simulink model "lane_dm6437_tcpip"  (Simulink 7.1)
settings: Solver=FixedStepDiscrete  SolverMode=SingleTasking  StartTime=0.0  StopTime=inf  RelTol=1e-3
PostLoadFcn:
  | NumRows=81
libraries: etargetslib x6, dspmtrx3 x2, viptransforms x2, dspindex x2, vipanalysis x1, vipobslib x1, dspstat3 x1, viptextngfix x1, vipstatistics x1, dspbioslib x1
CloseFcn:
  | clear vR3 vG3 vB3
settings Model: Creator=don  LastModifiedBy=Administrator
settings SolverCC: PositivePriorityOrder=on
settings DataIOCC: LimitDataPoints=off  SaveOutput=off  SaveTime=off  SignalLoggingName=sigsOut
settings OptimizationCC: EnforceIntegerDowncast=off  LocalBlockOutputs=off  OptimizeModelRefInitCode=on  BufferReusableBoundary=off
settings DebuggingCC: CheckExecutionContextPreStartOutputMsg=on  CheckExecutionContextRuntimeOutputMsg=on  SignalResolutionControl=TryResolveAllWithWarning  SolverPrmCheckMsg=none  MultiTaskDSMMsg=warning  MultiTaskCondExecSysMsg=none  SigSpecEnsureSampleTimeMsg=none
settings HardwareCC: ProdBitPerLong=40  ProdIntDivRoundTo=Zero  ProdEndianess=LittleEndian  ProdHWDeviceType=TI C6000  TargetHWDeviceType=32-bit Generic
settings ModelReferenceCC: UpdateModelReferenceTargets=IfOutOfDate
settings RTWCC: SystemTargetFile=ccslink_ert.tlc  GenerateMakefile=off  TemplateMakefile=ccslink_ert.tmf  Description=Embedded IDE Link CC (ERT) code generation for TMS320(TM) DSP platforms  ProcessScript=ccslink_ert_make_rtw_hook  IncludeERTFirstTime=on
settings CodeAppCC: IgnoreCustomStorageClasses=off
settings ERTTgtLinkCCS: TargetFcnLib=ansi_tfl_tmw_new.mat  TargetFunctionLibrary=ANSI_C  UtilityFuncGeneration=Auto  GenerateFullHeader=on  GenerateSampleERTMain=off  GenerateTestInterfaces=off  IsPILTarget=off  ModelReferenceCompliant=on  CompOptLevelCompliant=off  IncludeMdlTerminateFcn=on  CombineOutputUpdateFcns=on  SuppressErrorStatus=off  ERTFirstTimeCompliant=off  IncludeFileDelimiter=Auto  ERTCustomFileBanners=on  SupportAbsoluteTime=on  LogVarNameModifier=rt_  MatFileLogging=off  MultiInstanceERTCode=off  SupportNonFinite=on  SupportComplex=on  PurelyIntegerCode=off  SupportContinuousTime=off  SupportNonInlinedSFcns=off  EnableShiftOperators=on  ParenthesesLevel=Nominal  PortableWordSizes=off  ModelStepFunctionPrototypeControlCompliant=off  AutosarCompliant=off  GenerateErtSFunction=off  GenerateASAP2=off  ExtMode=off  ExtModeTransport=0  ExtModeStaticAlloc=on  ExtModeStaticAllocSize=1000000  ExtModeTesting=off  ExtModeMexFile=ext_comm  ExtModeIntrfLevel=Level1  InlinedParameterPlacement=NonHierarchical  TargetOS=BareBoardExample  MultiInstanceErrorCode=Error  RateGroupingCode=on  RootIOFormat=Individual arguments  RTWCAPISignals=off  RTWCAPIParams=off  RTWCAPIStates=off  ERTSrcFileBannerTemplate=ert_code_template.cgt  ERTHdrFileBannerTemplate=ert_code_template.cgt  ERTDataSrcFileTemplate=ert_code_template.cgt  ERTDataHdrFileTemplate=ert_code_template.cgt  ERTCustomFileTemplate=example_file_process.tlc  ModuleNamingRule=Unspecified  SignalDisplayLevel=10  ParamTuneLevel=10  GlobalDataDefinition=Auto  DataDefinitionFile=global.c  GlobalDataReference=Auto  DataReferenceFile=global.h  GRTInterface=off  PreserveExpressionOrder=off  PreserveIfCondition=off  EnableUserReplacementTypes=off  MemSecPackage=--- None ---  MemSecDataConstants=Default  MemSecDataIO=Default  MemSecDataInternal=Default  MemSecDataParameters=Default  MemSecFuncInitTerm=Default  MemSecFuncExecute=Default  exportIDEObj=on  ideObjName=CCS_Obj  oldideObjName=CCS_Obj  ideObjTimeout=10  oldideObjTimeout=10  ideObjBuildTimeout=1000  oldideObjBuildTimeout=1000  ProfileGenCode=off  ProfileNumSamples=100  InlineDSPBlks=on  projectOptions=Custom  debugCompilerOptions="-g -d\"_DEBUG\""  releaseCompilerOptions=-o2  customCompilerOptions=-o2 --mem_model:data=far  compilerOptionsStr=-o2 --mem_model:data=far  getCompilerOptions=off  getLinkerOptions=off  systemStackSize=8192  buildAction=Build  overrunNotificationMethod=None  overrunNotificationFcn=myfunction  oldoverrunNotificationFcn=myfunction  configurePIL=off  configPILBlockAction=None

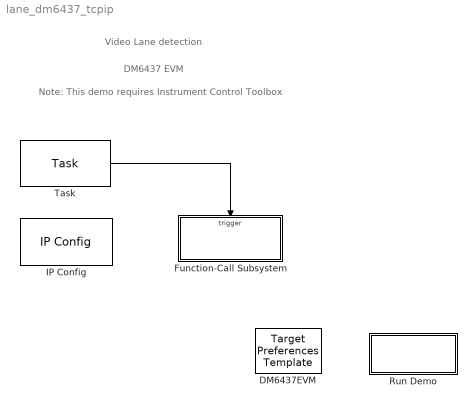
== system lane_dm6437_tcpip ==
  note: Video Lane detection
  note: DM6437 EVM
  note: Note: This demo requires Instrument Control Toolbox
  DM6437EVM : etargetslib/Target Preferences Template  Tag=ccslinktgtpref  SystemSampleTime=-1
  Function-Call Subsystem : Subsystem  TreatAsAtomicUnit=on
  IP Config : etargetslib/IP Config  boardType=DM6437EVM  daughterCard=Internal EMAC  tcpipStackDir=$(NDK_INSTALL_DIR)\packages\ti\ndk  enetIntNum=13  memSegment=DDR  enablePrintfs=on  dhcpEnabled=on  IPAddr=100.100.100.2  subnetMask=255.255.255.0  gatewayIP=100.100.100.1  dnsServerIP=0.0.0.0  domainName=mathworks.net  hostName=dm6437evm
  Run Demo : Subsystem  Description=Controls host-side RTDX processing.  AncestorBlock=demo_controls/Run Demo
      settings: OpenFcn=lane_tcpip_script('lane_pcl_tcpip');
      mask Display: disp(sprintf('Build / Reload\n& Run'))
  Task : dspbioslib/Task  SystemSampleTime=-1  taskName=Task0  taskPriority=1  taskExecutionOrder=1  taskStackSize=8192  stackMemSegment=IRAM  monitorStackUse=off  taskYield=off  parentmanaget=on  tickres=1/1000  ticklen=32bits  taskTrigger=off
  wires:
  Task/1 -> Function-Call Subsystem/Trigger

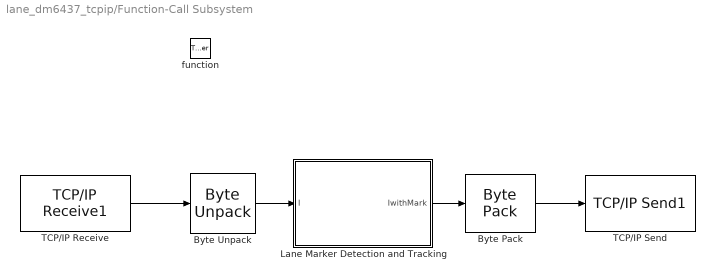
== system lane_dm6437_tcpip/Function-Call Subsystem ==
  function : TriggerPort  TriggerType=function-call
  Byte Pack : etargetslib/Byte Pack  datatypes={'uint8'}  byteAlign=1
  Byte Unpack : etargetslib/Byte Unpack  dimensions={[168, 360]}  datatypes={'uint8'}  byteAlign=1
  Lane Marker Detection and Tracking : Subsystem
  TCP/IP Receive : etargetslib/TCP//IP Receive1  connType=Server  remoteIf=0.0.0.0:0  localPort=49000  recvBuffSize=60480  enableBlockingMode=on  sampleTime=0.01  triggerType=Function call  dataSize=168*360  dataType=uint8  frameMode=Sample based
  TCP/IP Send : etargetslib/TCP//IP Send1  connType=Server  remoteIf=0.0.0.0:0  localPort=49000  sendBuffSize=60480
  wires:
  Byte Unpack/1 -> Lane Marker Detection and Tracking/1(I)
  TCP/IP Receive/1 -> Byte Unpack/1
  Byte Pack/1 -> TCP/IP Send/1
  Lane Marker Detection and Tracking/1(IwithMark) -> Byte Pack/1

== system lane_dm6437_tcpip/Run Demo ==

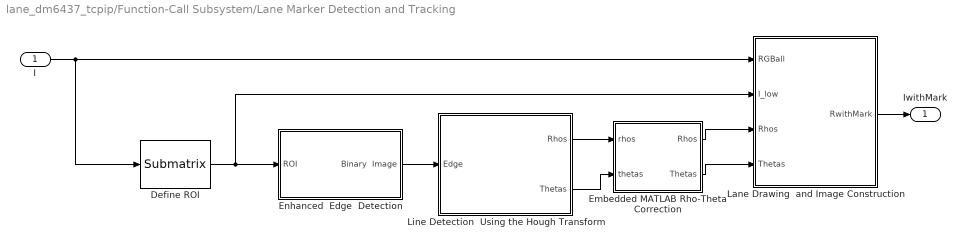
== system lane_dm6437_tcpip/Function-Call Subsystem/Lane Marker Detection and Tracking ==
  I : Inport  OutDataType=sfix(16)  OutScaling=2^0
  Define ROI : dspmtrx3/Submatrix  RowSpan=Range of rows  RowStartMode=Index  RowStartIndex=NumRows  RowEndMode=Last  RowEndIndex=1  ColSpan=All columns  ColStartMode=First  ColStartIndex=1  ColEndMode=Last  ColEndIndex=1
  Embedded MATLAB Rho-Theta Correction : Stateflow chart
  Enhanced  Edge  Detection : Subsystem
  Lane Drawing  and Image Construction : Subsystem
  Line Detection  Using the Hough Transform : Subsystem
  IwithMark : Outport  OutDataType=sfix(16)  OutScaling=2^0
  wires:
  I/1 -> Lane Drawing  and Image Construction/1(RGBall), Define ROI/1
  Lane Drawing  and Image Construction/1(RwithMark) -> IwithMark/1
  Enhanced  Edge  Detection/1(Binary  Image) -> Line Detection  Using the Hough Transform/1(Edge)
  Define ROI/1 -> Lane Drawing  and Image Construction/2(I_low), Enhanced  Edge  Detection/1(ROI)
  Line Detection  Using the Hough Transform/2(Thetas) -> Embedded MATLAB Rho-Theta Correction/2(thetas)
  Line Detection  Using the Hough Transform/1(Rhos) -> Embedded MATLAB Rho-Theta Correction/1(rhos)
  Embedded MATLAB Rho-Theta Correction/2(Thetas) -> Lane Drawing  and Image Construction/4(Thetas)
  Embedded MATLAB Rho-Theta Correction/1(Rhos) -> Lane Drawing  and Image Construction/3(Rhos)

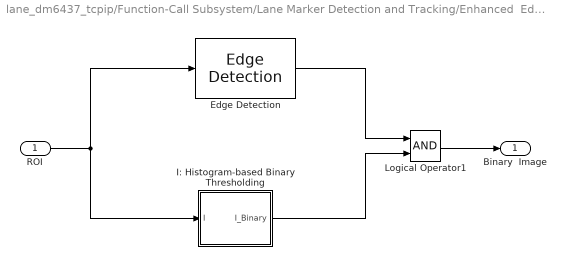
== system lane_dm6437_tcpip/Function-Call Subsystem/Lane Marker Detection and Tracking/Enhanced  Edge  Detection ==
  ROI : Inport  OutDataType=sfix(16)  OutScaling=2^0
  Edge Detection : vipanalysis/Edge Detection  DialogController=vipDDGCreate  DialogControllerArgs=DataTag1  method=Sobel  outputType=Binary image  userDefinedThreshold=off  thresholdSource=Input port  threshold=20  thresholdTuning=1  edgeThinning=off  threshold_canny=[0.25 0.60]  autoPercent=93  sigma=2  prodOutputMode=Binary point scaling  prodOutputWordLength=32  prodOutputFracLength=8  roundingMode=Floor  overflowMode=off
  I: Histogram-based Binary Thresholding : Subsystem
  Logical Operator1 : Logic  AllPortsSameDT=off  OutDataTypeMode=boolean  OutDataTypeStr=boolean
  Binary  Image : Outport  OutDataType=sfix(16)  OutScaling=2^0
  wires:
  I: Histogram-based Binary Thresholding/1(I_Binary) -> Logical Operator1/2
  Edge Detection/1 -> Logical Operator1/1
  ROI/1 -> Edge Detection/1, I: Histogram-based Binary Thresholding/1(I)
  Logical Operator1/1 -> Binary  Image/1

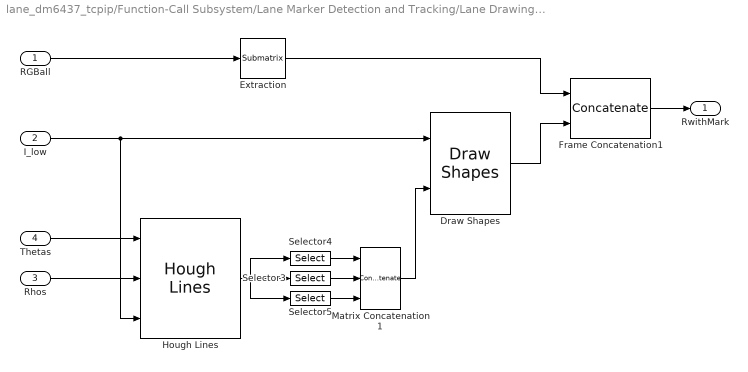
== system lane_dm6437_tcpip/Function-Call Subsystem/Lane Marker Detection and Tracking/Lane Drawing  and Image Construction ==
  RGBall : Inport  OutDataType=sfix(16)  OutScaling=2^0
  I_low : Inport  Port=2  OutDataType=sfix(16)  OutScaling=2^0
  Rhos : Inport  Port=3  OutDataType=sfix(16)  OutScaling=2^0
  Thetas : Inport  Port=4  OutDataType=sfix(16)  OutScaling=2^0
  Draw Shapes : viptextngfix/Draw Shapes  DialogController=vipDDGCreate  DialogControllerArgs=DataTag4  shape=Polygons  fill=on  display=User-specified value  intensity=200  color="[0  1 1]"  opacity=0.6  viewport=Entire image  antialiasing=on  inType=Intensity  imagePorts=One multidimensional signal
  Extraction : dspmtrx3/Submatrix  RowSpan=Range of rows  RowStartMode=First  RowStartIndex=50  RowEndMode=Index  RowEndIndex=NumRows-1  ColSpan=All columns  ColStartMode=First  ColStartIndex=1  ColEndMode=Last  ColEndIndex=1
  Frame Concatenation1 : Concatenate  Mode=Multidimensional array
  Hough Lines : viptransforms/Hough Lines  DialogController=vipDDGCreate  DialogControllerArgs=DataTag5  sineCompMethod=Trigonometric function  thetaRes=pi/180  firstCoeffMode=Specify word length  firstCoeffWordLength=16  firstCoeffFracLength=15  prodOutputMode=Binary point scaling  prodOutputWordLength=32  prodOutputFracLength=16  roundingMode=Nearest  overflowMode=on
  Matrix Concatenation1 : Concatenate  NumInputs=3  Mode=Multidimensional array
  Selector3 : Selector  NumberOfDimensions=2  InputPortWidth=3  IndexOptions=Index vector (dialog),Index vector (dialog)  Indices=3:4,2  OutputSizes=1
  Selector4 : Selector  NumberOfDimensions=2  InputPortWidth=3  IndexOptions=Select all,Index vector (dialog)  Indices=-1,1  OutputSizes=1
  Selector5 : Selector  NumberOfDimensions=2  InputPortWidth=3  IndexOptions=Index vector (dialog),Index vector (dialog)  Indices=1:2,2  OutputSizes=1
  RwithMark : Outport  OutDataType=sfix(16)  OutScaling=2^0
  wires:
  Extraction/1 -> Frame Concatenation1/1
  I_low/1 -> Draw Shapes/1, Hough Lines/3
  Thetas/1 -> Hough Lines/1
  Rhos/1 -> Hough Lines/2
  Frame Concatenation1/1 -> RwithMark/1
  Draw Shapes/1 -> Frame Concatenation1/2
  RGBall/1 -> Extraction/1
  Matrix Concatenation1/1 -> Draw Shapes/2
  Hough Lines/1 -> Selector5/1, Selector4/1, Selector3/1
  Selector5/1 -> Matrix Concatenation1/3
  Selector3/1 -> Matrix Concatenation1/2
  Selector4/1 -> Matrix Concatenation1/1

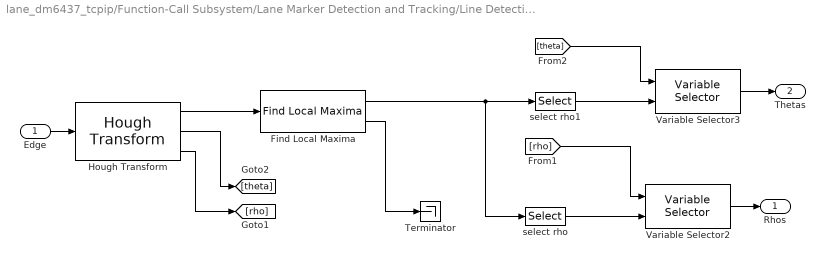
== system lane_dm6437_tcpip/Function-Call Subsystem/Lane Marker Detection and Tracking/Line Detection  Using the Hough Transform ==
  Edge : Inport  OutDataType=sfix(16)  OutScaling=2^0
  Find Local Maxima : vipstatistics/Find Local Maxima  num_peaks=2  nhood_size=[21 39]  src_thresh=Specify via dialog  threshold=10  inputIsHough=on  dt_peak=uint32  dt_count=uint32
  Hough Transform : viptransforms/Hough Transform  DialogController=vipDDGCreate  DialogControllerArgs=DataTag6  theta_res=pi/180  rho_res=2  out_theta_rho=on  outdtmode=single  firstCoeffMode=Binary point scaling  firstCoeffWordLength=16  firstCoeffFracLength=14  secondCoeffMode=Binary point scaling  secondCoeffWordLength=32  secondCoeffFracLength=16  outputMode=Binary point scaling  outputWordLength=16  outputFracLength=0  accumMode=Binary point scaling  accumWordLength=32  accumFracLength=20  prodOutputMode=Binary point scaling  prodOutputWordLength=32  prodOutputFracLength=20  memoryMode=Binary point scaling  memoryWordLength=32  memoryFracLength=16  roundingMode=Nearest  overflowMode=on
  Terminator : Terminator
  Variable Selector2 : dspindex/Variable Selector  NumInputs=1  rowsOrCols=Columns  IdxMode=Variable  Elements=[1 3]  ZerOneIdxMode=Zero-based  errmode=Clip Index  FillMode=on  FillValues=0
  Variable Selector3 : dspindex/Variable Selector  NumInputs=1  rowsOrCols=Columns  IdxMode=Variable  Elements=[1 3]  ZerOneIdxMode=Zero-based  errmode=Clip Index  FillMode=on  FillValues=0
  select rho : Selector  NumberOfDimensions=2  InputPortWidth=3  IndexOptions=Index vector (dialog),Select all  Indices=1,-1  OutputSizes=1
  select rho1 : Selector  NumberOfDimensions=2  InputPortWidth=3  IndexOptions=Index vector (dialog),Select all  Indices=2,-1  OutputSizes=1
  Rhos : Outport  OutDataType=sfix(16)  OutScaling=2^0
  Thetas : Outport  Port=2  OutDataType=sfix(16)  OutScaling=2^0
  wires:
  Find Local Maxima/2 -> Terminator/1
  Hough Transform/1 -> Find Local Maxima/1
  Edge/1 -> Hough Transform/1
  Variable Selector3/1 -> Thetas/1
  Variable Selector2/1 -> Rhos/1
  select rho1/1 -> Variable Selector3/2
  [theta] -> Variable Selector3/1
  Find Local Maxima/1 -> select rho1/1, select rho/1
  select rho/1 -> Variable Selector2/2
  [rho] -> Variable Selector2/1
  Hough Transform/2 -> [theta]
  Hough Transform/3 -> [rho]

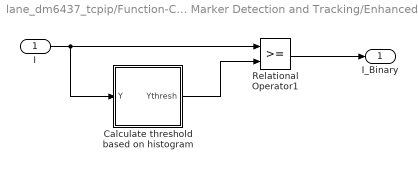
== system lane_dm6437_tcpip/Function-Call Subsystem/Lane Marker Detection and Tracking/Enhanced  Edge  Detection/I: Histogram-based Binary Thresholding ==
  I : Inport  OutDataType=sfix(16)  OutScaling=2^0
  Calculate threshold based on histogram : Subsystem
  Relational Operator1 : RelationalOperator  LogicOutDataTypeMode=boolean  OutDataTypeStr=boolean
  I_Binary : Outport  OutDataType=sfix(16)  OutScaling=2^0
  wires:
  Relational Operator1/1 -> I_Binary/1
  Calculate threshold based on histogram/1(Ythresh) -> Relational Operator1/2
  I/1 -> Calculate threshold based on histogram/1(Y), Relational Operator1/1

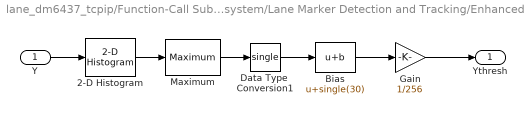
== system lane_dm6437_tcpip/Function-Call Subsystem/Lane Marker Detection and Tracking/Enhanced  Edge  Detection/I: Histogram-based Binary Thresholding/Calculate threshold based on histogram ==
  Y : Inport  OutDataType=sfix(16)  OutScaling=2^0
  2-D Histogram : vipobslib/2-D Histogram  DialogController=dspDDGCreate  DialogControllerArgs=DataTag2  umin=0  umax=1  nbins=256  normalized=off  run=off  reset=on  trigtype=Non-zero sample  operateOver=Entire input  Dimension=1  colComp=on  roundingMode=Floor  overflowMode=off
  Bias : Bias  Bias=single(30)
  Data Type  Conversion1 : DataTypeConversion  OutDataTypeMode=single  OutDataType=sfix(16)  OutScaling=2^0  OutDataTypeStr=single  SaturateOnIntegerOverflow=on  RndMeth=Zero
  Gain : Gain  Gain=1/256  ParameterDataType=sfix(16)  ParameterScaling=2^0  OutDataType=sfix(16)  OutScaling=2^0
  Maximum : dspstat3/Maximum  DialogController=dspfixptddg.MinMax  DialogControllerArgs=DataTag3  fcn=Index  reset=None  indexBase=One  operateOver=Each column  Dimension=1  colComp=on  operation=maximum  roundingMode=Floor  overflowMode=off
  Ythresh : Outport  OutDataType=sfix(16)  OutScaling=2^0
  wires:
  Gain/1 -> Ythresh/1
  Bias/1 -> Gain/1
  Data Type  Conversion1/1 -> Bias/1
  Maximum/1 -> Data Type  Conversion1/1
  2-D Histogram/1 -> Maximum/1
  Y/1 -> 2-D Histogram/1

== matlab function Function-Call Subsystem/Lane Marker Detection and Tracking/Embedded MATLAB Rho-Theta Correction ==
  data: rhos input double; Rhos output double; thetas input double; Thetas output double
function [Rhos, Thetas] = fcn(rhos, thetas)
% This block supports an embeddable subset of the MATLAB language.
% See the help menu for details.

%initialise a frame count
persistent count;
if isempty(count)
    count = 0;
end

%remember previous outputs
persistent lastRhos;
persistent lastThetas;

%initialise to same as first input for first entry into function
if isempty(lastRhos)
    lastRhos = rhos;
end
if isempty(lastThetas)
    lastThetas = thetas;
end


%Assume that all is OK initially
Rhos = rhos;
Thetas = thetas;


if count == 4
    %after the 4th frame, engage the test logic
    for I = 1:length(rhos)
        if (abs(rhos(I) - lastRhos(I)) > 30) || (abs(thetas(I) - lastThetas(I)) > 10*(pi/180))
            %too much change - just use the old values
%            outR(I) = lastRhos(I);
%            outT(I) = lastThetas(I);
            Rhos(I) = lastRhos(I);
            Thetas(I) = lastThetas(I);
        end
    end

else
    %otherwise just output the computed values
    count = count+1;
end

%assign outputs
%Rhos = outR;
%Thetas = outT;

%remember outputs for next time
lastRhos = Rhos;
lastThetas = Thetas;
